simulink model "generalBristleFriction2d_velocity_input"  (R2021b)
settings: Solver=VariableStepAuto  StartTime=0.0  StopTime=t_end  MaxStep=t_step  RelTol=1e-3  AbsTol=1e-3
values from neighbouring files (symbols this model uses):
  t_step = 0.001    [experiment_01_mass_variation.m]    (also in experiment_01_mass_variation_noslip.m; experiment_02_stick_slip_variation.m; experiment_03_lambda_variation.m; experiment_04_rheo_variation.m)
libraries: generalBristleFriction2d_lib x10, nesl_utility x2
settings Model: Creator=q657093  LastModifiedBy=Q657093
settings SolverCC: ZeroCrossAlgorithm=Adaptive
settings SimscapeCC: ExplicitSolverDiagnosticOptions=none  SimscapeLogType=all  SimscapeLogSimulationStatistics=on  SimscapeLogToSDI=on  SimscapeLogLimitData=off

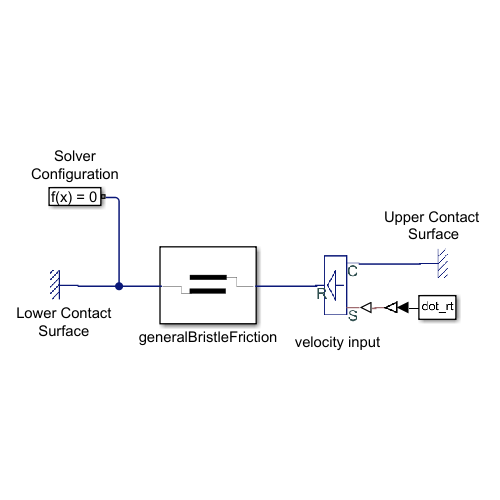
[thumbnail: Simulink's stored preview of the top-level diagram]
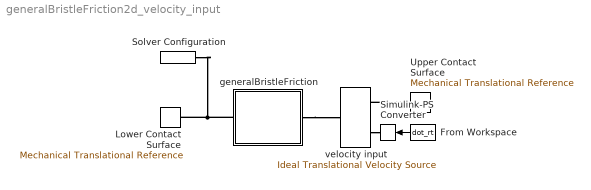
== system generalBristleFriction2d_velocity_input ==
  From Workspace : FromWorkspace  VariableName=dot_rt  SampleTime=t_step  OutputAfterFinalValue=Holding final value
  Lower Contact Surface : generalBristleFriction2d_lib/Mechanical Translational Reference
      settings: InternalSimscapePortConfiguration="{\"Bottom\":[],\"Left\":[{\"id\":\"V\",\"label\":\"\",\"type\":\"generalBristleFriction2d.translational2d\"}],\"Right\":[],\"Top\":[]}"
  Simulink-PS Converter : nesl_utility/Simulink-PS Converter  PhysicalDomain=network_engine_domain  SubClassName=ps_input  LeftPortType=input  RightPortType=output  PseudoPeriodic=off  Frequencies=[]  NoiseDistribution=none  NoiseParameters=[]  Unit=1  AffineConversion=off  FilteringAndDerivatives=provide  SimscapeFilterOrder=1  InputFilterTimeConstant=0.001  UdotUserProvided=0
      settings: SourceProductBaseCode=PW,SS
  Solver Configuration : nesl_utility/Solver Configuration  PhysicalDomain=network_engine_domain  SubClassName=solver  LeftPortType=input  RightPortType=generic  Tones=[]  Harmonics=[]  SimulateNoise=off  Profile=off  UseLocalSampling=off  EnableSwitchedLinearOptims=on  FrequencyDomain=off  UseCCode=off  RelTol=0.001  AbsTol=1e-06  MinStep=1e-09  ToWorkspace=off  RevertToSquareIcSolve=off  NumHomotopyIterations=100  PhasorMode=off  PhasorModeNumHarmonics=1  DoDC=off  ResidualTolerance=1e-09  UseLocalSolver=on  LocalSolverChoice=NE_BACKWARD_EULER_ADVANCER  LocalSolverSampleTime=t_step  DoFixedCost=off  MaxNonlinIter=3  MaxModeIter=2  ComputeImpulses=off  ImpulseIterations=2  LinearAlgebra=auto  EquationFormulation=NE_TIME_EF  DelaysMemoryBudget=1024  AutomaticFiltering=on  FilteringTimeConstant=t_step  PartitionStorageMethod=AS_NEEDED  PartitionMemoryBudget=1024  PartitionMethod=ROBUST
      settings: SourceProductBaseCode=PW,SS
  Upper Contact Surface : generalBristleFriction2d_lib/Mechanical Translational Reference
      settings: InternalSimscapePortConfiguration="{\"Bottom\":[],\"Left\":[{\"id\":\"V\",\"label\":\"\",\"type\":\"generalBristleFriction2d.translational2d\"}],\"Right\":[],\"Top\":[]}"
  generalBristleFriction : Subsystem
      mask Display: image('$imagefile'); % Use "Edit Image" on toolstrip to change.
  velocity input : generalBristleFriction2d_lib/Ideal Translational Velocity Source
      settings: InternalSimscapePortConfiguration="{\"Bottom\":[],\"Left\":[{\"id\":\"R\",\"label\":\"R\",\"type\":\"generalBristleFriction2d.translational2d\"}],\"Right\":[{\"id\":\"S\",\"label\":\"S\",\"type\":\"input\"},{\"id\":\"C\",\"label\":\"C\",\"type\":\"generalBristleFriction2d.translational2d\"}],\"Top\":[]}"
  wires:
  From Workspace/1 -> Simulink-PS Converter/1
  connections:
  Upper Contact Surface/LConn1 -- velocity input/RConn2
  Solver Configuration/RConn1 -- generalBristleFriction/LConn1 -- Lower Contact Surface/LConn1
  velocity input/RConn1 -- Simulink-PS Converter/RConn1
  generalBristleFriction/RConn1 -- velocity input/LConn1

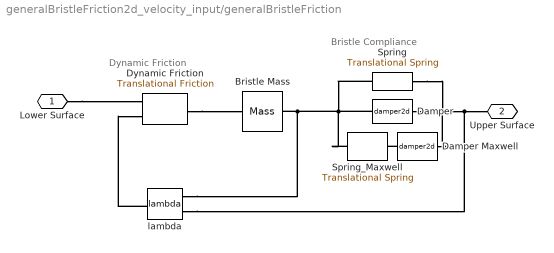
== system generalBristleFriction2d_velocity_input/generalBristleFriction ==
  note: Bristle Compliance
  note: Dynamic Friction
  Bristle Mass : generalBristleFriction2d_lib/Mass  mass=m_b kg  num_ports=foundation.enum.numPorts2.two  v_specify=off  v_priority=High  v=[0; 0] m/s  v_nominal_specify=off  v_nominal_unit=m/s  v_nominal_value=1  f_specify=off  f_priority=None  f=[0; 0] N  f_nominal_specify=off  f_nominal_unit=N  f_nominal_value=1
      settings: InternalSimscapePortConfiguration="{\"Bottom\":[],\"Left\":[{\"id\":\"M\",\"label\":\"\",\"type\":\"generalBristleFriction2d.translational2d\"}],\"Right\":[{\"id\":\"N\",\"label\":\"\",\"type\":\"generalBristleFriction2d.translational2d\"}],\"Top\":[]}"
  Damper : generalBristleFriction2d_lib/damper2d  dmp_rate=d N/(m/s)  v_specify=off  v_priority=None  v=[0; 0] m/s  v_nominal_specify=off  v_nominal_unit=m/s  v_nominal_value=1  f_specify=off  f_priority=None  f=[0; 0] N  f_nominal_specify=off  f_nominal_unit=N  f_nominal_value=1  x_specify=off  x_priority=High  x=[0; 0] m  x_nominal_specify=off  x_nominal_unit=m  x_nominal_value=1
      settings: InternalSimscapePortConfiguration="{\"Bottom\":[],\"Left\":[{\"id\":\"R\",\"label\":\"R\",\"type\":\"generalBristleFriction2d.translational2d\"}],\"Right\":[{\"id\":\"C\",\"label\":\"C\",\"type\":\"generalBristleFriction2d.translational2d\"}],\"Top\":[]}"
  Damper Maxwell : generalBristleFriction2d_lib/damper2d  dmp_rate=d_m N/(m/s)  v_specify=off  v_priority=None  v=[0; 0] m/s  v_nominal_specify=off  v_nominal_unit=m/s  v_nominal_value=1  f_specify=off  f_priority=None  f=[0; 0] N  f_nominal_specify=off  f_nominal_unit=N  f_nominal_value=1  x_specify=off  x_priority=High  x=[0; 0] m  x_nominal_specify=off  x_nominal_unit=m  x_nominal_value=1
      settings: InternalSimscapePortConfiguration="{\"Bottom\":[],\"Left\":[{\"id\":\"R\",\"label\":\"R\",\"type\":\"generalBristleFriction2d.translational2d\"}],\"Right\":[{\"id\":\"C\",\"label\":\"C\",\"type\":\"generalBristleFriction2d.translational2d\"}],\"Top\":[]}"
  Dynamic Friction : generalBristleFriction2d_lib/Translational Friction  F_g=F_g N  F_h=F_h N  v_minslip=v_minslip m/s  lambda_flag=lambda_flag  v_specify=off  v_priority=None  v=[0; 0] m/s  v_nominal_specify=off  v_nominal_unit=m/s  v_nominal_value=1  f_specify=off  f_priority=None  f=[0; 0] N  f_nominal_specify=off  f_nominal_unit=N  f_nominal_value=1  stick_specify=on  stick_priority=None  stick=1
      settings: InternalSimscapePortConfiguration="{\"Bottom\":[],\"Left\":[{\"id\":\"R\",\"label\":\"R\",\"type\":\"generalBristleFriction2d.translational2d\"}],\"Right\":[{\"id\":\"C\",\"label\":\"C\",\"type\":\"generalBristleFriction2d.translational2d\"},{\"id\":\"lambda\",\"label\":\"lambda\",\"type\":\"input\"}],\"Top\":[]}"
  Spring : generalBristleFriction2d_lib/Translational Spring  spr_rate=k N/m  v_specify=off  v_priority=None  v=[0; 0] m/s  v_nominal_specify=off  v_nominal_unit=m/s  v_nominal_value=1  f_specify=off  f_priority=None  f=[0; 0] N  f_nominal_specify=off  f_nominal_unit=N  f_nominal_value=1  x_specify=off  x_priority=High  x=[0; 0] m  x_nominal_specify=off  x_nominal_unit=m  x_nominal_value=1
      settings: InternalSimscapePortConfiguration="{\"Bottom\":[],\"Left\":[{\"id\":\"R\",\"label\":\"R\",\"type\":\"generalBristleFriction2d.translational2d\"}],\"Right\":[{\"id\":\"C\",\"label\":\"C\",\"type\":\"generalBristleFriction2d.translational2d\"}],\"Top\":[]}"
  Spring_Maxwell : generalBristleFriction2d_lib/Translational Spring  spr_rate=k_m N/m  v_specify=off  v_priority=None  v=[0; 0] m/s  v_nominal_specify=off  v_nominal_unit=m/s  v_nominal_value=1  f_specify=off  f_priority=None  f=[0; 0] N  f_nominal_specify=off  f_nominal_unit=N  f_nominal_value=1  x_specify=off  x_priority=High  x=[0; 0] m  x_nominal_specify=off  x_nominal_unit=m  x_nominal_value=1
      settings: InternalSimscapePortConfiguration="{\"Bottom\":[],\"Left\":[{\"id\":\"R\",\"label\":\"R\",\"type\":\"generalBristleFriction2d.translational2d\"}],\"Right\":[{\"id\":\"C\",\"label\":\"C\",\"type\":\"generalBristleFriction2d.translational2d\"}],\"Top\":[]}"
  lambda : generalBristleFriction2d_lib/lambda  F_g=F_g N  lambda_flag=lambda_flag
      settings: InternalSimscapePortConfiguration="{\"Bottom\":[],\"Left\":[{\"id\":\"top\",\"label\":\"t\",\"type\":\"generalBristleFriction2d.translational2d\"},{\"id\":\"bottom\",\"label\":\"b\",\"type\":\"generalBristleFriction2d.translational2d\"}],\"Right\":[{\"id\":\"l\",\"label\":\"l\",\"type\":\"output\"}],\"Top\":[]}"
  Lower Surface : PMIOPort  Side=Left
  Upper Surface : PMIOPort  Port=2  Side=Right
  connections:
  lambda/RConn1 -- Dynamic Friction/RConn2
  Dynamic Friction/LConn1 -- Bristle Mass/RConn1
  Lower Surface/RConn1 -- Dynamic Friction/RConn1
  lambda/LConn2 -- Spring_Maxwell/RConn1 -- Spring/RConn1 -- Damper/RConn1 -- Bristle Mass/LConn1
  Damper/LConn1 -- Spring/LConn1 -- Damper Maxwell/LConn1 -- lambda/LConn1 -- Upper Surface/RConn1
  Damper Maxwell/RConn1 -- Spring_Maxwell/LConn1
